simulink model "MultirotorSimPx4"  (R2018b)
settings: Solver=VariableStepAuto  StartTime=0.0  StopTime=Simulation.T_END  MaxStep=Simulation.TS_MAX  RelTol=1e-3  EnableMultiTasking=on
PreLoadFcn:
  | % InitializeParameters;
undefined symbols (not defined in the file): Aero, Initial, Motor, Simulation, Uav
libraries: QuaternionLibrary x13, simulink_extras x9, Px4Library x4, simulink x1
(part 1 of 8)
settings Model: Creator=jban039  LastModifiedBy=jban039
settings DataIOCC: Decimation=10  ReturnWorkspaceOutputs=on  OutputOption=SpecifiedOutputTimes  OutputTimes=Simulation.T_OUT
settings OptimizationCC: LifeSpan=inf
settings DebuggingCC: ReadBeforeWriteMsg=DisableAll  WriteAfterWriteMsg=DisableAll  WriteAfterReadMsg=DisableAll  MultiTaskDSMMsg=none  UnconnectedLineMsg=none  AllowSymbolicDim=off  SFUnexpectedBacktrackingDiag=warning  SFNoUnconditionalDefaultTransitionDiag=warning  SFExecutionAtInitializationDiag=none
settings ModelReferenceCC: UpdateModelReferenceTargets=IfOutOfDate  ModelReferenceMinAlgLoopOccurrences=on  PropagateSignalLabelsOutOfModel=off
settings SFSimCC: SFSimEcho=off  SimUseLocalCustomCode=off
settings RTWCC: RTWUseLocalCustomCode=off
settings CodeAppCC: StateflowObjectComments=on
settings GRTTargetCC: TargetLangStandard=C89/C90 (ANSI)
settings ConfigComp: CovMetricSettings=dw  CovHtmlReporting=on  CovSaveCumulativeToWorkspaceVar=on  CovSaveSingleToWorkspaceVar=on  CovExternalEMLEnable=off

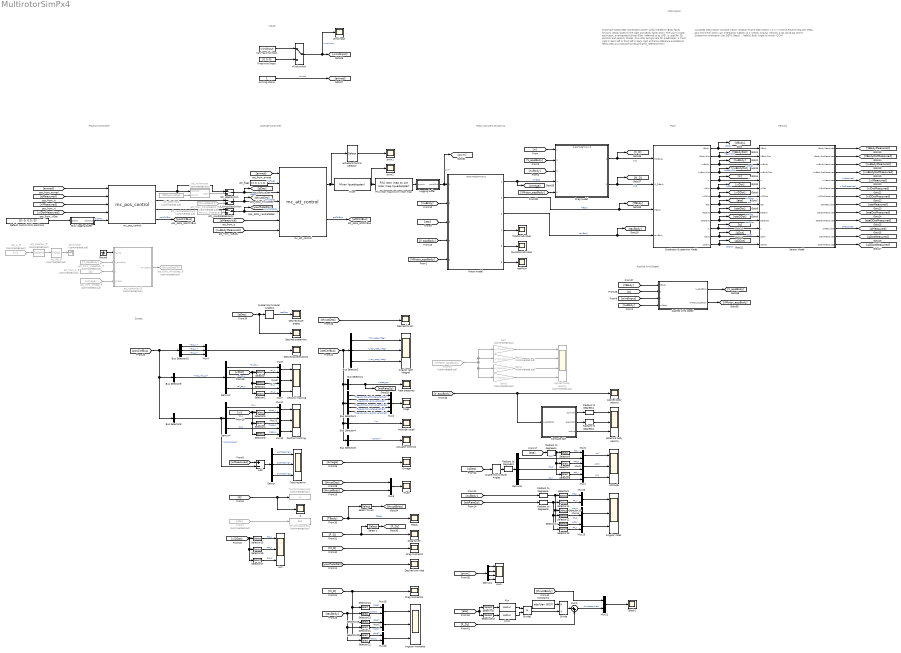
== system MultirotorSimPx4 ==
  note: Important Notes
      |
      | NED coordinate system used, therefore xBody faces forward, yBody faces to the right and zBody faces down.
      | The UAV's state estimator, an extended kalman filter (referred to as LPE), is used for 3D position and velocity states.
      | PX4 rotor assignment for quadcopter:
      | 1: front right
      | 2: back left
      | 3: front left
      | 4: back right
      | Airframe reference available at:
      | https://dev.px4.io/en/airframes/airframe_reference.html
  note: Variables Description
      |
      | Variable
      | Vector notation
      | Frame
      | Description
      |
      | xi
      | [x y z]
      | World
      | Position
      |
      | eta
      | [phi theta psi]
      | World
      | Roll pitch yaw orientation
      |
      | nuBody
      | [p q r]
      | Body
      | Angular velocity
      |
      | q
      | [q1 q2 q3 q4]
      | World
      | Quaternion orientation
      |
      | Uav.BETA
      | [beta1 ... betaN]
      | Body
      | Angle to motor (CCW)
  note: Applied Wind Speed
  note: Inputs
  note: Scopes
  note: Information
  note: Plant
  note: Motor and Aero Dynamics
  note: Sensors
  note: Attitude Controller
  note: Position Controller
  Acc : Scope  NumInputPorts=3
  Actuator controls : Scope
  Add : Sum  Inputs=+-
  Angular moments : Scope  NumInputPorts=3
  Angular rate integral : Scope  NumInputPorts=3
  Angular rates : Scope  NumInputPorts=3
  Applied body velocity : Scope
  Applied motor velocity : Scope  Commented=on  NumInputPorts=4
  Applied wind speed : Subsystem
  Arming status : Constant
  Attitude : Scope  NumInputPorts=3
  Attitude (quat) : Scope
  Bus Selector1 : BusSelector  OutputSignals=rates_sp
  Bus Selector10 : BusSelector  OutputSignals=mpc_local_pos_sp.acc_x,mpc_local_pos_sp.acc_y,mpc_local_pos_sp.acc_z
  Bus Selector2 : BusSelector  OutputSignals=controller_status.roll_rate_integ,controller_status.pitch_rate_integ,controller_status.yaw_rate_integ
  Bus Selector3 : BusSelector  OutputSignals=v_control_mode.flag_control_attitude_enabled,v_control_mode.flag_control_auto_enabled,v_control_mode.flag_control_manual_enabled,v_control_mode.flag_control_rates_enabled,v_control_mode.flag_control_velocity_enabled
  Bus Selector4 : BusSelector  OutputSignals=ctrl_state.q
  Bus Selector6 : BusSelector  OutputSignals=actuators.control
  Bus Selector8 : BusSelector  OutputSignals=mpc_pos_sp
  Bus Selector9 : BusSelector  OutputSignals=mpc_vel_sp
  Compute Sph : MATLAB Function  TreatAsAtomicUnit=on
  Constant1 : Constant  Value=abs(Uav.G(3))
  Default control stick positions : Constant  Value=[0; 0; 0.5; 0]
  Demux{,2,4,6} (4 alike) : Demux  Outputs=3
  Demux1 : Demux
  Desired accelerations : Scope
  Desired euler angles : Scope
  Desired quaternion : Scope
  Desired thrust : Scope
  Desired yaw rate : Scope
  Divide : Product  Inputs=*/
  Divide1 : Product  Inputs=**
  Drag forces : Scope
  Drag model : ModelReference  ModelNameDialog=DragModelAIAAv3  SimulationMode=Normal  ModelReferenceVersion=1.368
  Drag moments : Scope
  Drag moments1 : Scope
  Fcn : Fcn  Expr=cos(u)
  Fcn1 : Fcn  Expr=cos(u)
  Fixed wind input : Constant  Value=[0 0 0]
  Flags : Scope
  From37 : From  Commented=on  GotoTag=VMotor_appBody
  From7 : From  Commented=on  GotoTag=eta
  Gain : Gain  Commented=on  Gain=[1;0;0;0]  Multiplication=Matrix(u*K)
  Gain1 : Gain  Commented=on  Gain=[0;1;0;0]  Multiplication=Matrix(u*K)
  Gain2 : Gain  Commented=on  Gain=[0;0;1;0]  Multiplication=Matrix(u*K)
  Gain3 : Gain  Commented=on  Gain=[0;0;0;1]  Multiplication=Matrix(u*K)
  Ground : Ground
  Logging buffer : Subsystem
  Mixer : Px4Library/Mixer (quadcopter)  MC_SAMPLING_PERIOD=0.002
  Motor model : ModelReference  ModelNameDialog=MotorModelAIAAv3  SimulationMode=Normal  ModelReferenceVersion=1.397
  Mux{1,3,5..18,21} (17 alike) : Mux  Inputs=2
  Mux2 : Mux  Inputs=5
  Mux4 : Mux  Inputs=3
  Omega : Scope
  PX4 rotor map to sim rotor map : Px4Library/PX4 rotor map to sim rotor map (quadcopter)  SystemSampleTime=-1
  Position tracking : Scope  NumInputPorts=3
  Quadrotor Quaternion Model : Subsystem
  Quaternion to Euler Angles : QuaternionLibrary/Quaternion to Euler Angles
  Quaternion to Euler Angles1 : QuaternionLibrary/Quaternion to Euler Angles
  Radians to Degrees{1..6} (6 alike) : simulink_extras/Transformations/Radians to Degrees
  Rate setpoints : Scope
  Select Thrust : Selector  InputPortWidth=3  IndexOptions=Index vector (dialog)  Indices=[3]  OutputSizes=1
  Select pitch : Selector  InputPortWidth=3  IndexOptions=Index vector (dialog)  Indices=2  OutputSizes=1
  Select roll : Selector  InputPortWidth=3  IndexOptions=Index vector (dialog)  Indices=1  OutputSizes=1
  Select z : Selector  InputPortWidth=3  IndexOptions=Index vector (dialog)  Indices=[3]  OutputSizes=1
  Selector{,3,6,9,14..15,23..24} (8 alike) : Selector  InputPortWidth=3  IndexOptions=Index vector (dialog)  Indices=1  OutputSizes=1
  Selector{1,4,7,10,12,16,19,21} (8 alike) : Selector  InputPortWidth=3  IndexOptions=Index vector (dialog)  Indices=2  OutputSizes=1
  Selector{2,5,8,11,13,17,20,22} (8 alike) : Selector  InputPortWidth=3  IndexOptions=Index vector (dialog)  Indices=3  OutputSizes=1
  Sensor Model : Subsystem
  Spherical body velocity : Scope  NumInputPorts=3
  Stick logging buffer : Subsystem
  Sum3 : Sum  Inputs=|++
  TBody : Scope
  TBody1 : Scope
  TMotorIndividual : Scope
  Terminator : Terminator  Commented=on
  Thust : Scope
  To Workspace eta : ToWorkspace  Commented=on  VariableName=eta  SaveFormat=Structure With Time  SampleTime=0.01
  To Workspace quat : ToWorkspace  Commented=on  VariableName=q  SaveFormat=Structure With Time  SampleTime=0.01
  Tracking error : Scope  NumInputPorts=3
  Varying wind input : FromWorkspace  VariableName=windInput  SampleTime=0
  Velocity tracking : Scope  NumInputPorts=3
  Wind Input : Scope
  Wind switch : ManualSwitch
  actuatorsControl selector : Selector  InputPortWidth=8  IndexOptions=Index vector (dialog)  Indices=[1 2 3]  OutputSizes=1
  att_Goto_thrustDes_ff : Goto  Commented=on  GotoTag=thrustDesFF
  att_PID_ff : simulink/Continuous/PID Controller  Commented=on  Controller=PID  Form=Parallel  TimeDomain=Continuous-time  SampleTime=-1  IntegratorMethod=Forward Euler  FilterMethod=Forward Euler  ControllerParametersSource=internal  P=-22.065410118279  I=-10.2297340963903  D=-11.7817329577601  UseFilter=on  N=104.897155810233  TunerSelectOption=Transfer Function Based (PID Tuner App)  InitialConditionSource=internal  InitialConditionForIntegrator=0  InitialConditionForFilter=0  DifferentiatorICPrevScaledInput=0  ExternalReset=none  TrackingMode=off  Kt=1  LimitOutput=off  UpperSaturationLimit=inf  LowerSaturationLimit=-inf  LinearizeAsGain=on  AntiWindupMode=none  Kb=1  POutMin=[]  POutMax=[]  IOutMin=[]  IOutMax=[]  DOutMin=[]  DOutMax=[]  NOutMin=[]  NOutMax=[]  SumOutMin=[]  SumOutMax=[]  SaturationOutMin=[]  SaturationOutMax=[]  PParamMin=[]  PParamMax=[]  IParamMin=[]  IParamMax=[]  DParamMin=[]  DParamMax=[]  NParamMin=[]  NParamMax=[]  KbParamMin=[]  KbParamMax=[]  KtParamMin=[]  KtParamMax=[]  KbOutMin=[]  KbOutMax=[]  KtOutMin=[]  KtOutMax=[]  IntegratorOutMin=[]  IntegratorOutMax=[]  FilterOutMin=[]  FilterOutMax=[]  SumI1OutMin=[]  SumI1OutMax=[]  SumI2OutMin=[]  SumI2OutMax=[]  SumI3OutMin=[]  SumI3OutMax=[]  SumI4OutMin=[]  SumI4OutMax=[]  SumDOutMin=[]  SumDOutMax=[]  DifferentiatorOutMin=[]  DifferentiatorOutMax=[]  FilterDiffOutCoefMin=[]  FilterDiffOutCoefMax=[]  ReciprocalOutMin=[]  ReciprocalOutMax=[]  SumDenOutMin=[]  SumDenOutMax=[]  SumNumOutMin=[]  SumNumOutMax=[]  DivideOutMin=[]  DivideOutMax=[]  IntegratorContinuousStateAttributes=''  IntegratorStateMustResolveToSignalObject=off  IntegratorRTWStateStorageClass=Auto  FilterContinuousStateAttributes=''  FilterStateMustResolveToSignalObject=off  FilterRTWStateStorageClass=Auto  ParallelPVariant=InternalParameters  IdealPVariant=Disabled  IVariant=InternalParameters  DVariant=InternalParameters  IntegratorVariant=Continuous  SatVariant=Disabled  AWVariant=Passthrough  PCopyVariant=Disabled  TRVariant=Disabled  FdbkBlocksVariant=Forward  IdealPFdbkVariant=Disabled  SatFdbkVariant=Disabled  DerivativeFilterVariant=ContFilter  NVariant=InternalParameters  NCopyVariant=Disabled  FilterICVariant=InternalICsFilter  IntegratorICVariant=InternalICs  ExternalResetVariant=Disabled  TRSumVariant=Passthrough  SumFdbkVariant=Disabled  SumVariant=Sum_PID
  att_controller_ff : MATLAB Function  Commented=on  TreatAsAtomicUnit=on
  att_flags : Constant  Value=[1, 0, 1, 1, 1]
  att_from_VappBody_ff : From  Commented=on  GotoTag=V_appBody
  att_from_omega_ff : From  Commented=on  GotoTag=omega
  att_from_q_ff : From  Commented=on  GotoTag=q
  att_from_thrustDesFF_ff : From  Commented=on  GotoTag=thrustDesFF
  att_mixerInput : Subsystem  Commented=on
  att_qDesInput : FromWorkspace  Commented=on  VariableName=AttInput.qDes  SampleTime=0  Interpolate=off  OutputAfterFinalValue=Holding final value
  att_qDesSwitch : ManualSwitch
  att_selector_ff : Selector  Commented=on  InputPortWidth=3  IndexOptions=Index vector (dialog)  Indices=3  OutputSizes=1
  att_thrustDesSwitch : ManualSwitch
  att_xi_ff : From  Commented=on  GotoTag=xi
  att_yawRateDesInput : FromWorkspace  Commented=on  VariableName=AttInput.yawRateDes  SampleTime=0  Interpolate=off  OutputAfterFinalValue=Holding final value
  att_yawRateDesSwitch : ManualSwitch
  mc_att_control : Px4Library/mc_att_control  MC_SAMPLING_PERIOD=0.004  MC_ROLL_TC=0.2  MC_PITCH_TC=0.2  MC_ROLL_P=6.5  MC_ROLLRATE_P=0.15  MC_ROLLRATE_I=0.05  MC_ROLLRATE_D=0.003  MC_ROLLRATE_FF=0  MC_PITCH_P=6.5  MC_PITCHRATE_P=0.15  MC_PITCHRATE_I=0.05  MC_PITCHRATE_D=0.003  MC_PITCHRATE_FF=0.0  MC_YAW_P=2.8  MC_YAWRATE_P=0.2  MC_YAWRATE_I=0.1  MC_YAWRATE_D=0.0  MC_YAWRATE_FF=0.0  MC_YAW_FF=0.5  MC_ROLLRATE_MAX=220.0  MC_PITCHRATE_MAX=220.0  MC_YAWRATE_MAX=200.0  MC_YAWRAUTO_MAX=45.0  MC_ACRO_R_MAX=360.0  MC_ACRO_P_MAX=360.0  MC_ACRO_Y_MAX=360.0  MC_RATT_TH=1.0  MC_TPA_BREAK=1.0  MC_TPA_SLOPE=1.0  VT_OPT_RECOV_EN=0.0  VT_WV_YAWR_SCL=0.15  MC_RR_INT_LIM=0.30  MC_PR_INT_LIM=0.30  MC_TPA_BREAK_P=1.0  MC_TPA_BREAK_I=1.0  MC_TPA_BREAK_D=1.0  MC_TPA_RATE_P=0.0  MC_TPA_RATE_I=0.0  MC_TPA_RATE_D=0.0  VT_TYPE=2  MC_BAT_SCALE_EN=0  MC_YR_INT_LIM=0.30
  mc_pos_control : Px4Library/mc_pos_control  THROTTLE_HOVER=Uav.THROTTLE_HOVER  MPC_SAMPLING_PERIOD=0.02  MPC_THR_MIN=0.120  MPC_THR_HOVER=0.500  MPC_ALTCTL_DZ=0.100  MPC_ALTCTL_DY=0.0  MPC_THR_MAX=0.900  MPC_MANTHR_MIN=0.080  MPC_MANTHR_MAX=0.900  MPC_Z_P=1.000  MPC_Z_VEL_P=0.200  MPC_Z_VEL_I=0.020  MPC_Z_VEL_D=0.0  MPC_Z_VEL_MAX_UP=3.0  MPC_Z_VEL_MAX=1.000  MPC_Z_VEL_MAX_DN=1.000  MPC_Z_FF=0.500  MPC_XY_P=0.950  MPC_XY_VEL_P=0.090  MPC_XY_VEL_I=0.020  MPC_XY_VEL_D=0.010  MPC_XY_CRUISE=5.0  MPC_XY_VEL_MAX=8.0  MPC_XY_FF=0.500  MPC_TILTMAX_AIR=45.0  MPC_TILTMAX_LND=12.0  MPC_LAND_SPEED=0.500  MPC_TKO_SPEED=1.500  MPC_MAN_R_MAX=35.0  MPC_MAN_P_MAX=35.0  MPC_MAN_Y_MAX=200.0  MPC_HOLD_XY_DZ=0.100  MPC_HOLD_MAX_XY=0.800  MPC_HOLD_MAX_Z=0.600  MPC_VELD_LP=5.0  MPC_ACC_HOR_MAX=5.0  MPC_ALT_MODE=0.0  MC_YAWRATE_MAX=200.0  MC_YAW_P=2.8  VT_OPT_RECOV_EN=0.0
  pwm : Scope  NumInputPorts=4
  pwm1 : Scope
  pwm2 : Scope
  q : Scope
  realPwm : Scope
  tauMotorIndividual : Scope
  wires:
  Motor model/1 -> [omega], Drag model/4  "omega"
  Motor model/2 -> Quadrotor Quaternion Model/3(TBody), [TBody]  "TBody"
  Drag model/2 -> Quadrotor Quaternion Model/2(M_DBody), [M_D]  "M_D"
  Quadrotor Quaternion Model/1(VBody) -> Sensor Model/1(VBody), [VBody]  "VBody"
  Quadrotor Quaternion Model/2(VBodyDot) -> Sensor Model/2(VBodyDot), [VBodyDot]  "VBodyDot"
  Quadrotor Quaternion Model/3(nuBody) -> Sensor Model/3(nuBody), [nuBody]  "nuBody"
  Quadrotor Quaternion Model/4(nuBodyDot) -> Sensor Model/4(nuBodyDot), [nuBodyDot]  "nuBodyDot"
  Quadrotor Quaternion Model/5(xi) -> Sensor Model/5(xi), [xi]  "xi"
  Quadrotor Quaternion Model/6(xiDot) -> Sensor Model/6(xiDot), [xiDot]  "xiDot"
  Quadrotor Quaternion Model/7(xiDDot) -> Sensor Model/7(xiDDot), [xiDDot]  "xiDDot"
  Quadrotor Quaternion Model/8(eta) -> Sensor Model/8(eta), [eta]  "eta"
  Quadrotor Quaternion Model/9(etaDot) -> Sensor Model/9(etaDot), [etaDot]  "etaDot"
  Quadrotor Quaternion Model/10(etaDDot) -> Sensor Model/10(etaDDot), [etaDDot]  "etaDDot"
  [V_appBody] -> Drag model/2
  [nuBody] -> Motor model/2
  Quadrotor Quaternion Model/11(q) -> Sensor Model/11(q), [q]  "q"
  Quadrotor Quaternion Model/12(qDot) -> Sensor Model/12(qDot), [qDot]  "qDot"
  Quadrotor Quaternion Model/13(qDDot) -> Sensor Model/13(qDDot), [qDDot]  "qDDot"
  Drag model/1 -> Quadrotor Quaternion Model/1(F_DBody), [F_D]  "F_D"
  Sensor Model/1(VBodyMeasured) -> [VBodyMeasured]
  Sensor Model/2(VBodyDotMeasured) -> [VBodyDotMeasured]
  Sensor Model/3(nuBodyMeasured) -> [nuBodyMeasured]
  Sensor Model/4(nuBodyDotMeasured) -> [nuBodyDotMeasured]
  Sensor Model/5(xiMeasured) -> [xiMeasured]  "xiMeasured"
  Sensor Model/6(xiDotMeasured) -> [xiDotMeasured]  "xiDotMeasured"
  Sensor Model/7(xiDDotMeasured) -> [xiDDotMeasured]
  Sensor Model/8(etaMeasured) -> [etaMeasured]
  Sensor Model/9(etaDotMeasured) -> [etaDotMeasured]
  Sensor Model/10(etaDDotMeasured) -> [etaDDotMeasured]
  Sensor Model/11(qMeasured) -> [qMeasured]  "qMeasured"
  Sensor Model/12(qDotMeasured) -> [qDotMeasured]
  Sensor Model/13(qDDotMeasured) -> [qDDotMeasured]
  Logging buffer/1(pwmOut) -> [pwm], Motor model/1  "pwm"
  Bus Selector2/1 -> Angular rate integral/1  "<roll_rate_integ>"
  Bus Selector2/2 -> Angular rate integral/2  "<pitch_rate_integ>"
  Bus Selector2/3 -> Angular rate integral/3  "<yaw_rate_integ>"
  [attCtrlBus] -> Bus Selector2/1, Bus Selector1/1, Bus Selector6/1, Bus Selector4/1, Bus Selector3/1
  Bus Selector1/1 -> [attRateSp], Rate setpoints/1  "<rates_sp>"
  Bus Selector3/1 -> Mux2/1  "<flag_control_attitude_enabled>"
  Bus Selector3/2 -> Mux2/2  "<flag_control_auto_enabled>"
  Bus Selector3/3 -> Mux2/3  "<flag_control_manual_enabled>"
  Bus Selector3/4 -> Mux2/4  "<flag_control_rates_enabled>"
  Bus Selector3/5 -> Mux2/5  "<flag_control_velocity_enabled>"
  Mux2/1 -> Flags/1
  Bus Selector4/1 -> Attitude (quat)/1  "<q>"
  Bus Selector6/1 -> Actuator controls/1  "<control>"
  [posCtrlBus] -> Bus Selector10/1, Bus Selector9/1, Bus Selector8/1
  Stick logging buffer/1(stickOut) -> mc_pos_control/5  "stickPos"
  [qMeasured] -> mc_att_control/6
  [nuBodyMeasured] -> mc_att_control/7
  [qMeasured] -> mc_pos_control/2
  mc_pos_control/3 -> att_yawRateDesSwitch/1
  att_controller_ff/1(thrustDes) -> att_Goto_thrustDes_ff/1
  Bus Selector9/1 -> Demux2/1  "<mpc_vel_sp>"
  [xiDotMeasured] -> mc_pos_control/4
  [xiMeasured] -> mc_pos_control/3
  Bus Selector10/1 -> Mux4/1  "<acc_x>"
  Bus Selector10/2 -> Mux4/2  "<acc_y>"
  Bus Selector10/3 -> Mux4/3  "<acc_z>"
  Mux4/1 -> Desired accelerations/1
  Selector6/1 -> Mux6/1  "act_r"
  Selector7/1 -> Mux5/1  "act_p"
  Mux7/1 -> Velocity tracking/3
  Mux8/1 -> Velocity tracking/2
  Mux9/1 -> Velocity tracking/1
  Demux2/1 -> Mux9/1  "vel_sp_x"
  Selector/1 -> Mux9/2  "vel_x"
  Demux2/2 -> Mux8/1  "vel_sp_y"
  Selector1/1 -> Mux8/2  "vel_y"
  Demux2/3 -> Mux7/1  "vel_sp_z"
  Selector2/1 -> Mux7/2  "vel_z"
  Mux10/1 -> Position tracking/3
  Mux11/1 -> Position tracking/2
  Mux12/1 -> Position tracking/1
  Demux4/1 -> Mux12/1  "sp_x"
  Selector3/1 -> Mux12/2  "meas_x"
  Demux4/2 -> Mux11/1  "sp_y"
  Selector4/1 -> Mux11/2  "meas_y"
  Demux4/3 -> Mux10/1  "sp_z"
  Selector5/1 -> Mux10/2  "meas_z"
  Quaternion to Euler Angles/1 -> Radians to Degrees3/1
  Demux6/1 -> Mux6/2  "sp_r"
  Demux6/2 -> Mux5/2  "sp_p"
  Demux6/3 -> Mux1/2  "sp_y"
  Selector8/1 -> Mux1/1  "act_y"
  [qDes] -> Quaternion to Euler Angles/1
  Mixer/1 -> pwm2/1, PX4 rotor map to sim rotor map/1
  PX4 rotor map to sim rotor map/1 -> Logging buffer/1(pwmIn)
  Bus Selector8/1 -> Add/2, Demux4/1  "<mpc_pos_sp>"
  Add/1 -> Demux/1
  Demux/1 -> Tracking error/1  "posTrackingX"
  Demux/2 -> Tracking error/2  "posTrackingY"
  Demux/3 -> Tracking error/3  "posTrackingZ"
  [nuBody] -> Drag model/3
  Mux6/1 -> Attitude/1  "roll"
  Mux5/1 -> Attitude/2  "pitch"
  [eta] -> Motor model/3
  [q] -> q/1, To Workspace quat/1
  From7/1 -> To Workspace eta/1
  [xiDot] -> Selector2/1, Selector1/1, Selector/1
  [xi] -> Selector5/1, Selector4/1, Selector3/1
  [xiMeasured] -> Add/1
  Wind switch/1 -> [windInput], Wind Input/1  "windInput"
  [V_appBody] -> Motor model/4
  att_flags/1 -> mc_att_control/2  "mcFlags"
  Arming status/1 -> [armed]  "armed"
  mc_pos_control/4 -> [posCtrlBus]  "posCtrlBus"
  mc_att_control/2 -> [attCtrlBus]  "attCtrlBus"
  [armed] -> mc_att_control/1
  [armed] -> mc_pos_control/1
  Fixed wind input/1 -> Wind switch/2
  Varying wind input/1 -> Wind switch/1
  [omega] -> Omega/1
  Radians to Degrees3/1 -> Demux6/1
  Radians to Degrees4/1 -> Selector8/1, Selector7/1, Selector6/1
  [eta] -> Radians to Degrees4/1
  Motor model/4 -> TMotorIndividual/1
  [thrustDes] -> Mux3/1
  [thrustBody] -> Mux3/2
  Mux3/1 -> Thust/1
  Motor model/5 -> tauMotorIndividual/1
  [xi] -> Drag model/1
  [TBody] -> Select Thrust/1, TBody/1  "TBody"
  Select Thrust/1 -> [thrustBody]
  [F_D] -> Drag forces/1, Select z/1
  [V_appBody] -> Compute Sph/1(V_appBody), Applied body velocity/1
  Compute Sph/1(azimuth) -> Radians to Degrees1/1
  Compute Sph/2(elevation) -> Radians to Degrees2/1
  Compute Sph/3(radius) -> Spherical body velocity/3
  Radians to Degrees1/1 -> Spherical body velocity/1
  Radians to Degrees2/1 -> Spherical body velocity/2
  [M_D] -> Drag moments/1
  [VMotor_appBody] -> Motor model/5
  From37/1 -> Gain3/1, Gain2/1, Gain/1, Gain1/1
  Gain/1 -> Applied motor velocity/1
  Gain1/1 -> Applied motor velocity/2
  Gain2/1 -> Applied motor velocity/3
  Gain3/1 -> Applied motor velocity/4
  [VMotor_appBody] -> Drag model/5
  att_qDesSwitch/1 -> [qDes], mc_att_control/3  "qDes"
  att_thrustDesSwitch/1 -> [thrustDes], mc_att_control/4  "thrustDes"
  att_yawRateDesSwitch/1 -> [yawRateDes], mc_att_control/5  "yawRateDes"
  att_yawRateDesInput/1 -> att_yawRateDesSwitch/2
  att_from_thrustDesFF_ff/1 -> att_thrustDesSwitch/2
  [yawRateDes] -> Desired yaw rate/1
  Mux1/1 -> Attitude/3  "yaw"
  Motor model/3 -> Quadrotor Quaternion Model/4(tauBody), [tauBody]  "tauBody"
  [VBody] -> Applied wind speed/1(VBody)
  [q] -> Applied wind speed/2(q)
  [windInput] -> Applied wind speed/3(U)
  Applied wind speed/1(V_appBody) -> [V_appBody]
  Applied wind speed/2(VMotor_appBody) -> [VMotor_appBody]
  [nuBody] -> Applied wind speed/4(nuBody)
  Selector9/1 -> Mux15/1  "act_r"
  Selector10/1 -> Mux14/1  "act_p"
  Selector11/1 -> Mux13/1  "act_y"
  Mux15/1 -> Angular rates/1
  Mux14/1 -> Angular rates/2
  Radians to Degrees5/1 -> Selector9/1, Selector11/1, Selector10/1
  [nuBody] -> Radians to Degrees5/1
  Mux13/1 -> Angular rates/3
  Radians to Degrees6/1 -> Selector14/1, Selector13/1, Selector12/1
  Selector14/1 -> Mux15/2  "sp_r"
  Selector12/1 -> Mux14/2  "sp_p"
  Selector13/1 -> Mux13/2  "sp_y"
  [attRateSp] -> Radians to Degrees6/1
  Selector15/1 -> Acc/1  "acc_x"
  Selector16/1 -> Acc/2  "acc_y"
  Selector17/1 -> Acc/3  "acc_z"
  [xiDDot] -> Selector15/1, Selector16/1, Selector17/1
  [thrustDes] -> Desired thrust/1
  actuatorsControl selector/1 -> pwm1/1
  [M_D] -> Selector20/1, Selector19/1, Selector24/1, Drag moments1/1
  Mux18/1 -> Angular moments/1
  Mux17/1 -> Angular moments/2
  Mux16/1 -> Angular moments/3
  Selector24/1 -> Mux18/1  "dragX"
  Selector23/1 -> Mux18/2  "motorX"
  Selector19/1 -> Mux17/1  "dragY"
  Selector21/1 -> Mux17/2  "motorY"
  Selector20/1 -> Mux16/1  "dragZ"
  Selector22/1 -> Mux16/2  "MotorZ"
  [tauBody] -> Selector22/1, Selector21/1, Selector23/1
  Default control stick positions/1 -> Stick logging buffer/1(stickIn)
  [qDes] -> Desired quaternion/1, Quaternion to Euler Angles1/1
  Quaternion to Euler Angles1/1 -> Desired euler angles/1  "etaDes"
  att_from_VappBody_ff/1 -> att_controller_ff/2(V_appBody)
  att_selector_ff/1 -> att_PID_ff/1
  att_xi_ff/1 -> att_selector_ff/1
  att_from_q_ff/1 -> att_controller_ff/3(q)
  att_from_omega_ff/1 -> att_controller_ff/4(omega)
  Divide/1 -> Sum3/1
  Sum3/1 -> Mux21/2  "thrustRequired"
  Mux21/1 -> TBody1/1
  Constant1/1 -> Divide/1
  Select z/1 -> [F_Dz]
  [thrustBody] -> Mux21/1
  [eta] -> Select pitch/1, Select roll/1
  Select roll/1 -> Fcn/1
  Select pitch/1 -> Fcn1/1
  Fcn/1 -> Divide1/1
  Fcn1/1 -> Divide1/2
  Divide1/1 -> Divide/2
  [F_Dz] -> Sum3/2
  mc_pos_control/1 -> att_qDesSwitch/1, att_mixerInput/1(qPosCtrl)
  mc_pos_control/2 -> att_thrustDesSwitch/1
  att_mixerInput/1(qDes) -> att_qDesSwitch/2
  att_qDesInput/1 -> att_mixerInput/2(qInput)
  att_PID_ff/1 -> Terminator/1
  Ground/1 -> att_controller_ff/1(Textra)
  [pwm] -> Demux1/1
  Demux1/1 -> pwm/1
  Demux1/2 -> pwm/2
  Demux1/3 -> pwm/3
  Demux1/4 -> pwm/4
  Motor model/6 -> realPwm/1
  mc_att_control/1 -> actuatorsControl selector/1, Mixer/1

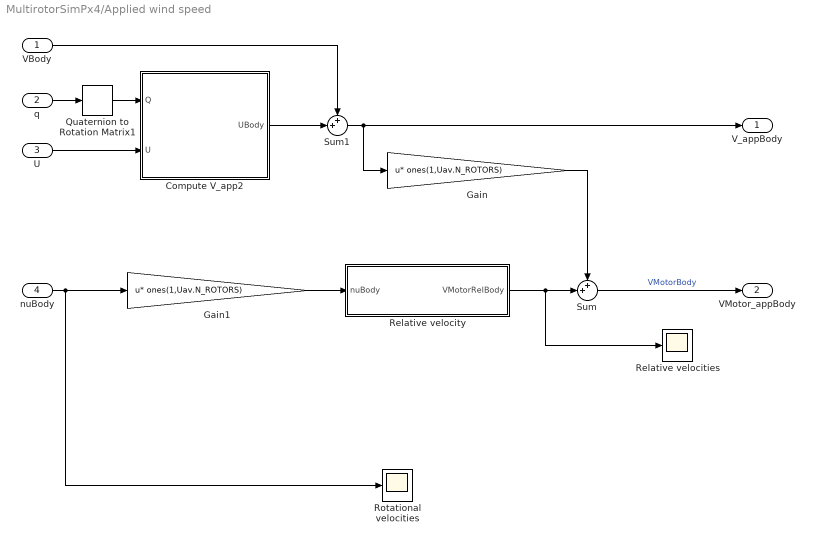
== system MultirotorSimPx4/Applied wind speed ==
  VBody : Inport  Unit=m/s
  q : Inport  Port=2
  U : Inport  Port=3  Unit=m/s
  nuBody : Inport  Port=4  Unit=rad/s
  Compute V_app2 : MATLAB Function  TreatAsAtomicUnit=on
  Gain : Gain  Gain=ones(1,Uav.N_ROTORS)  Multiplication=Matrix(u*K)
  Gain1 : Gain  Gain=ones(1,Uav.N_ROTORS)  Multiplication=Matrix(u*K)
  Quaternion to Rotation Matrix1 : QuaternionLibrary/Quaternion to Rotation Matrix
  Relative velocities : Scope
  Relative velocity : MATLAB Function  TreatAsAtomicUnit=on
  Rotational velocities : Scope
  Sum : Sum  Inputs=++|
  Sum1 : Sum  Inputs=++|
  V_appBody : Outport  Unit=m/s
  VMotor_appBody : Outport  Port=2  Unit=m/s  PortDimensions=[3,Uav.N_ROTORS]
  wires:
  U/1 -> Compute V_app2/2(U)
  Sum/1 -> VMotor_appBody/1  "VMotorBody"
  Quaternion to Rotation Matrix1/1 -> Compute V_app2/1(Q)
  nuBody/1 -> Gain1/1, Rotational velocities/1
  Gain/1 -> Sum/1
  VBody/1 -> Sum1/1
  q/1 -> Quaternion to Rotation Matrix1/1
  Relative velocity/1(VMotorRelBody) -> Relative velocities/1, Sum/2
  Compute V_app2/1(UBody) -> Sum1/2
  Sum1/1 -> Gain/1, V_appBody/1
  Gain1/1 -> Relative velocity/1(nuBody)

== system MultirotorSimPx4/Logging buffer ==
  pwmIn : Inport
  Rate Transition : RateTransition
  pwmOut : Outport
  wires:
  pwmIn/1 -> Rate Transition/1
  Rate Transition/1 -> pwmOut/1

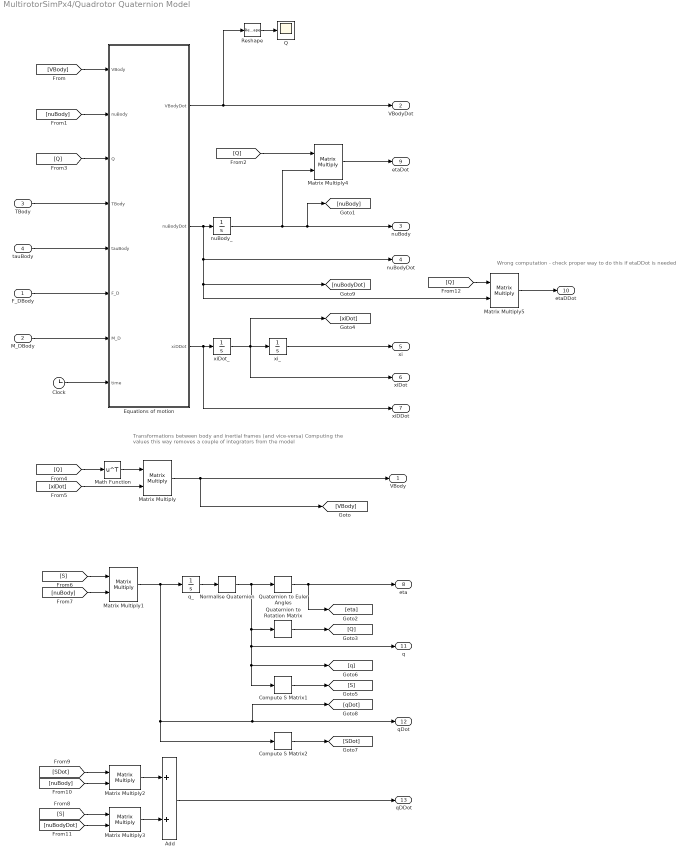
== system MultirotorSimPx4/Quadrotor Quaternion Model ==
  note: Wrong computation - check proper way to do this if etaDDot is needed
  note: Transformations between body and inertial frames (and vice-versa)
      | Computing the values this way removes a couple of integrators from the model
  F_DBody : Inport  Unit=N
  M_DBody : Inport  Port=2  Unit=N*m
  TBody : Inport  Port=3  Unit=N
  tauBody : Inport  Port=4  Unit=N*m
  Add : Sum
  Clock : Clock
  Compute S Matrix1 : QuaternionLibrary/Compute S Matrix
  Compute S Matrix2 : QuaternionLibrary/Compute S Matrix
  Equations of motion : MATLAB Function  TreatAsAtomicUnit=on
  Math Function : Math  Operator=transpose  SaturateOnIntegerOverflow=on
  Matrix Multiply{,1..5} (6 alike) : Product  Multiplication=Matrix(*)
  Normalise Quaternion : QuaternionLibrary/Normalise Quaternion
  Q : Scope
  Quaternion to Euler Angles : QuaternionLibrary/Quaternion to Euler Angles
  Quaternion to Rotation Matrix : QuaternionLibrary/Quaternion to Rotation Matrix
  Reshape : Reshape  OutputDimensionality=Column vector (2-D)
  nuBody_ : Integrator  InitialCondition=Initial.NU_BODY
  q_ : Integrator  InitialCondition=Initial.Q
  xiDot_ : Integrator  InitialCondition=Initial.XI_DOT
  xi_ : Integrator  InitialCondition=Initial.XI
  VBody : Outport  Unit=m/s
  VBodyDot : Outport  Port=2  Unit=m/s^2
  nuBody : Outport  Port=3  Unit=rad/s
  nuBodyDot : Outport  Port=4  Unit=rad/s^2
  xi : Outport  Port=5  Unit=m
  xiDot : Outport  Port=6  Unit=m/s
  xiDDot : Outport  Port=7  Unit=m/s^2
  eta : Outport  Port=8  Unit=rad
  etaDot : Outport  Port=9  Unit=rad/s
  etaDDot : Outport  Port=10  Unit=rad/s^2
  q : Outport  Port=11
  qDot : Outport  Port=12
  qDDot : Outport  Port=13
  wires:
  Equations of motion/1(VBodyDot) -> Reshape/1, VBodyDot/1
  xi_/1 -> xi/1
  [nuBody] -> Equations of motion/2(nuBody)
  [VBody] -> Equations of motion/1(VBody)
  tauBody/1 -> Equations of motion/5(tauBody)
  TBody/1 -> Equations of motion/4(TBody)
  Equations of motion/3(xiDDot) -> xiDot_/1, xiDDot/1
  F_DBody/1 -> Equations of motion/6(F_D)
  Matrix Multiply/1 -> VBody/1, [VBody]
  M_DBody/1 -> Equations of motion/7(M_D)
  nuBody_/1 -> Matrix Multiply4/2, [nuBody], nuBody/1
  Equations of motion/2(nuBodyDot) -> nuBody_/1, nuBodyDot/1, Matrix Multiply5/2, [nuBodyDot]
  q_/1 -> Normalise Quaternion/1
  Quaternion to Euler Angles/1 -> eta/1, [eta]
  Matrix Multiply4/1 -> etaDot/1
  Quaternion to Rotation Matrix/1 -> [Q]
  [Q] -> Equations of motion/3(Q)
  [Q] -> Math Function/1
  [xiDot] -> Matrix Multiply/2
  Math Function/1 -> Matrix Multiply/1
  [S] -> Matrix Multiply1/1
  [nuBody] -> Matrix Multiply1/2
  Compute S Matrix2/1 -> [SDot]
  [S] -> Matrix Multiply3/1
  Matrix Multiply1/1 -> qDot/1, [qDot], Compute S Matrix2/1, q_/1
  [SDot] -> Matrix Multiply2/1
  [nuBody] -> Matrix Multiply2/2
  [nuBodyDot] -> Matrix Multiply3/2
  Matrix Multiply2/1 -> Add/1
  Matrix Multiply3/1 -> Add/2
  Normalise Quaternion/1 -> Quaternion to Euler Angles/1, q/1, Compute S Matrix1/1, [q], Quaternion to Rotation Matrix/1
  Compute S Matrix1/1 -> [S]
  [Q] -> Matrix Multiply4/1
  Add/1 -> qDDot/1
  [Q] -> Matrix Multiply5/1
  Matrix Multiply5/1 -> etaDDot/1
  Reshape/1 -> Q/1
  xiDot_/1 -> xi_/1, [xiDot], xiDot/1
  Clock/1 -> Equations of motion/8(time)
